simulink model "FM_whisle"  (Simulink 7.8)
settings: Solver=ode45  StartTime=0.0  StopTime=2  RelTol=1e-3
libraries: commsynccomp2 x1, dspsnks4 x1
settings Model: Creator=morelos_zaragoza  LastModifiedBy=morelos_zaragoza
settings OptimizationCC: InlineInvariantSignals=on  InitFltsAndDblsToZero=on
settings DebuggingCC: SaveWithParameterizedLinksMsg=none  SignalResolutionControl=TryResolveAllWithWarning  MultiTaskDSMMsg=warning  MultiTaskCondExecSysMsg=none  StrictBusMsg=None
settings RTWCC: IncludeERTFirstTime=on
settings GRTTargetCC: TargetFcnLib=ansi_tfl_tmw.mat

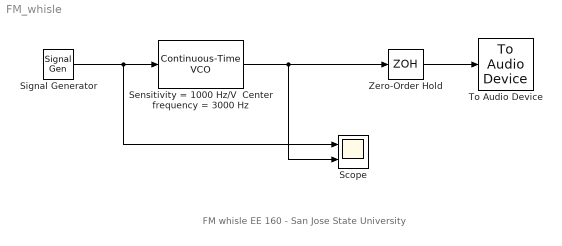
== system FM_whisle ==
  note: FM whisle
      | EE 160 - San Jose State University
  Scope : Scope  NumInputPorts=2
      settings: TimeRange=0.01  YMin=-1.5~-5  YMax=1.5~5
  Sensitivity = 1000 Hz/V  Center frequency = 3000 Hz : commsynccomp2/Continuous-Time VCO  Ac=3  Fc=3000  Kc=1000  Ph=0
  Signal Generator : SignalGenerator  Frequency=2
  To Audio Device : dspsnks4/To Audio Device  deviceName=Default  inheritSampleRate=off  sampleRate=16000  deviceDatatype=Determine from input data type  autoBufferSize=off  bufferSize=512  queueDuration=0.1
  Zero-Order Hold : ZeroOrderHold  SampleTime=1/44100
  wires:
  Signal Generator/1 -> Sensitivity = 1000 Hz/V  Center frequency = 3000 Hz/1, Scope/1
  Sensitivity = 1000 Hz/V  Center frequency = 3000 Hz/1 -> Scope/2, Zero-Order Hold/1
  Zero-Order Hold/1 -> To Audio Device/1
